simulink model "RC_Modelling"  (R2024a)
settings: Solver=FixedStepAuto  StartTime=0.0  StopTime=300  FixedStep=0.001  RelTol=1e-3
settings Model: Creator=devendra  LastModifiedBy=devendra

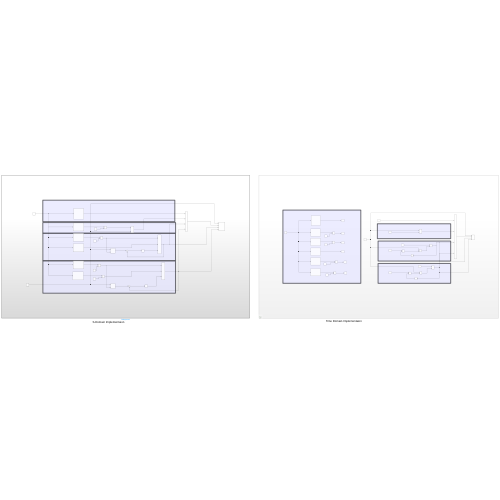
[thumbnail: Simulink's stored preview of the top-level diagram]
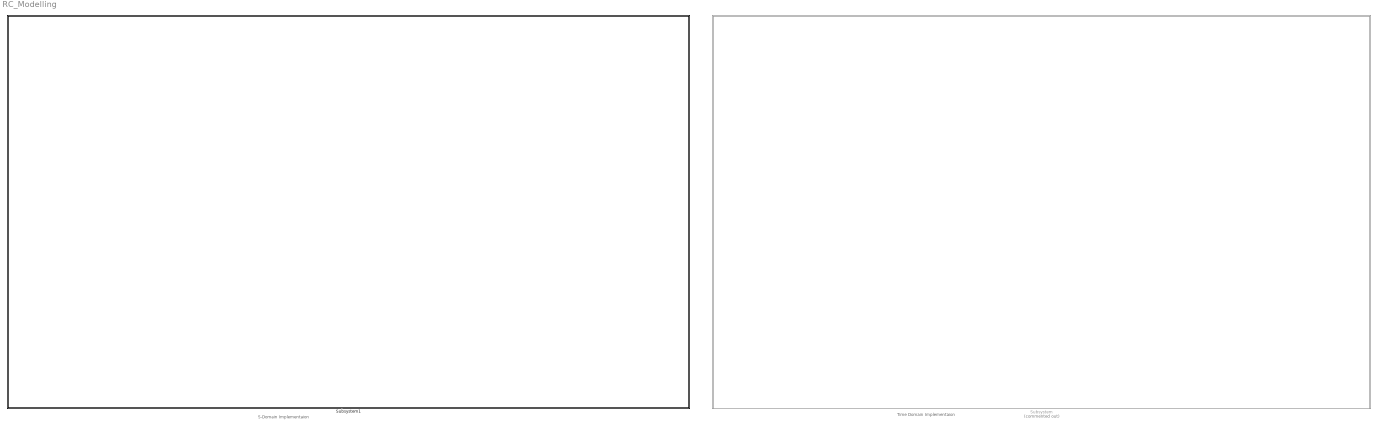
== system RC_Modelling ==
  note: Time Domain Implementaion
  note: S-Domain Implementaion
  Subsystem : Subsystem  Commented=on
  Subsystem1 : Subsystem

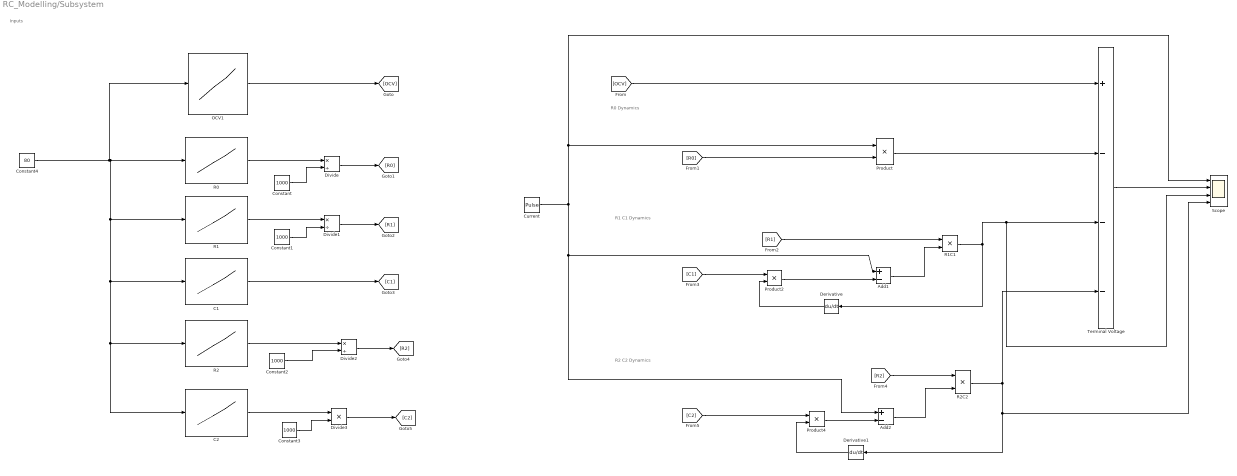
== system RC_Modelling/Subsystem ==
  note: Inputs
  note: R0 Dynamics
  note: R2 C2 Dynamics
  note: R1 C1 Dynamics
  Add1 : Sum  Inputs=+-
  Add2 : Sum  Inputs=+-
  C1 : Lookup_n-D  NumberOfTableDimensions=1  BreakpointsForDimension1=[0 5 10 20 30 40 50 60 70 80 90 100]  Table=[248 1482.7 2404.3 2466.7 2383.2 2193 2154.8 1498.3 1300.3 1714.9 1725.1 1840]  InternalRulePriority=Speed  RndMeth=Simplest
  C2 : Lookup_n-D  NumberOfTableDimensions=1  BreakpointsForDimension1=[0 5 10 20 30 40 50 60 70 80 90 100]  Table=[20.5 144.6 103 56.8 94.3 228 199.5 65.5 23.3 19.4 143 151]  InternalRulePriority=Speed  RndMeth=Simplest
  Constant{,1..3} (4 alike) : Constant  Value=1000
  Constant4 : Constant  Value=80
  Current : DiscretePulseGenerator  PulseType=Time based  Amplitude=5  Period=300  PulseWidth=25  SampleTime=100
  Derivative : Derivative
  Derivative1 : Derivative
  Divide : Product  Inputs=*/
  Divide1 : Product  Inputs=*/
  Divide2 : Product  Inputs=*/
  Divide3 : Product  Inputs=**
  OCV1 : Lookup_n-D  NumberOfTableDimensions=1  BreakpointsForDimension1=[0 5 10 15 20 30 40 50 60 70 80 90 95 100]  Table=[3.45 3.48 3.53 3.58 3.6 3.63 3.68 3.78 3.88 3.94 4.01 4.08 4.12 4.19]  InternalRulePriority=Speed  RndMeth=Simplest
  Product : Product
  Product2 : Product
  Product4 : Product
  R0 : Lookup_n-D  NumberOfTableDimensions=1  BreakpointsForDimension1=[0 5 10 20 30 40 50 60 70 80 90 100]  Table=[116.9 49 43.2 39.3 38.5 38.1 37.6 37.1 37 37.3 38.8 39]  InternalRulePriority=Speed  RndMeth=Simplest
  R1 : Lookup_n-D  NumberOfTableDimensions=1  BreakpointsForDimension1=[0 5 10 20 30 40 50 60 70 80 90 100]  Table=[67.5 22.6 21.6 25.8 22.4 20.2 21.6 22.2 19.8 20.8 23 23.7]  InternalRulePriority=Speed  RndMeth=Simplest
  "R1C1 " : Product
  R2 : Lookup_n-D  NumberOfTableDimensions=1  BreakpointsForDimension1=[0 5 10 20 30 40 50 60 70 80 90 100]  Table=[14.2 4.3 5.3 11.2 5.9 3.4 7.7 19 16.9 12.8 3.4 5]  InternalRulePriority=Speed  RndMeth=Simplest
  R2C2 : Product
  Scope : Scope  NumInputPorts=4
  Terminal Voltage : Sum  Inputs=+---
  wires:
  Product4/1 -> Add2/2
  Product/1 -> Terminal Voltage/2
  Add1/1 -> "R1C1 "/2
  "R1C1 "/1 -> Derivative/1, Scope/3, Terminal Voltage/3
  R2C2/1 -> Terminal Voltage/4, Scope/4, Derivative1/1
  Product2/1 -> Add1/2
  Current/1 -> Add2/1, Add1/1, Scope/1, Product/1
  [C1] -> Product2/1
  [R1] -> "R1C1 "/1
  Derivative/1 -> Product2/2
  [R2] -> R2C2/1
  Terminal Voltage/1 -> Scope/2
  Derivative1/1 -> Product4/2
  [C2] -> Product4/1
  [OCV] -> Terminal Voltage/1
  Add2/1 -> R2C2/2
  [R0] -> Product/2
  OCV1/1 -> [OCV]
  R0/1 -> Divide/1
  Constant/1 -> Divide/2
  R1/1 -> Divide1/1
  Constant1/1 -> Divide1/2
  Constant2/1 -> Divide2/2
  C2/1 -> Divide3/1
  Constant3/1 -> Divide3/2
  Divide/1 -> [R0]
  Divide1/1 -> [R1]
  C1/1 -> [C1]
  Divide2/1 -> [R2]
  Divide3/1 -> [C2]
  R2/1 -> Divide2/1
  Constant4/1 -> OCV1/1, C2/1, R2/1, C1/1, R1/1, R0/1

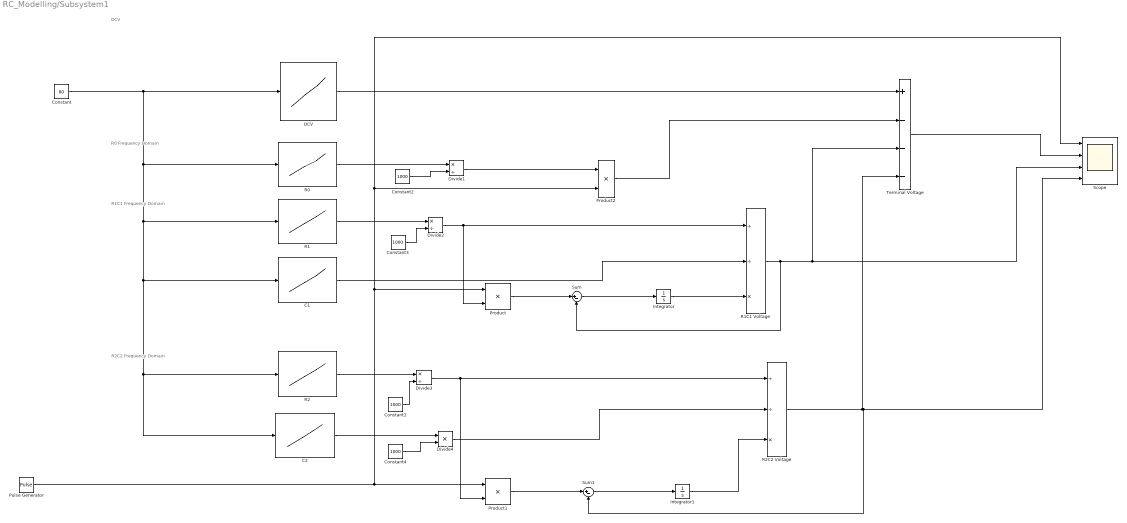
== system RC_Modelling/Subsystem1 ==
  note: R2C2 Frequency Domain
  note: R1C1 Frequency Domain
  note: R0 Frequency Domain
  note: OCV
  C1 : Lookup_n-D  NumberOfTableDimensions=1  BreakpointsForDimension1=[0 5 10 20 30 40 50 60 70 80 90 100]  Table=[248 1482.7 2404.3 2466.7 2383.2 2193 2154.8 1498.3 1300.3 1714.9 1725.1 1840]  InternalRulePriority=Speed  RndMeth=Simplest
  C2 : Lookup_n-D  NumberOfTableDimensions=1  BreakpointsForDimension1=[0 5 10 20 30 40 50 60 70 80 90 100]  Table=[20.5 144.6 103 56.8 94.3 228 199.5 65.5 23.3 19.4 143 151]  InternalRulePriority=Speed  RndMeth=Simplest
  Constant : Constant  Value=80
  Constant{1..4} (4 alike) : Constant  Value=1000
  Divide1 : Product  Inputs=*/
  Divide2 : Product  Inputs=*/
  Divide3 : Product  Inputs=*/
  Divide4 : Product  Inputs=**
  Integrator : Integrator
  Integrator1 : Integrator
  OCV : Lookup_n-D  NumberOfTableDimensions=1  BreakpointsForDimension1=[0 5 10 15 20 30 40 50 60 70 80 90 95 100]  Table=[3.45 3.48 3.53 3.58 3.6 3.63 3.68 3.78 3.88 3.94 4.01 4.08 4.12 4.19]  InternalRulePriority=Speed  RndMeth=Simplest
  Product : Product
  Product1 : Product
  Product2 : Product
  Pulse Generator : DiscretePulseGenerator  PulseType=Time based  Amplitude=5  Period=300  PulseWidth=25
  R0 : Lookup_n-D  NumberOfTableDimensions=1  BreakpointsForDimension1=[0 5 10 20 30 40 50 60 70 80 90 100]  Table=[116.9 49 43.2 39.3 38.5 38.1 37.6 37.1 37 37.3 38.8 39]  InternalRulePriority=Speed  RndMeth=Simplest
  R1 : Lookup_n-D  NumberOfTableDimensions=1  BreakpointsForDimension1=[0 5 10 20 30 40 50 60 70 80 90 100]  Table=[67.5 22.6 21.6 25.8 22.4 20.2 21.6 22.2 19.8 20.8 23 23.7]  InternalRulePriority=Speed  RndMeth=Simplest
  R1C1 Voltage : Product  Inputs=//*
  R2 : Lookup_n-D  NumberOfTableDimensions=1  BreakpointsForDimension1=[0 5 10 20 30 40 50 60 70 80 90 100]  Table=[14.2 4.3 5.3 11.2 5.9 3.4 7.7 19 16.9 12.8 3.4 5]  InternalRulePriority=Speed  RndMeth=Simplest
  R2C2 Voltage : Product  Inputs=//*
  Scope : Scope  NumInputPorts=4
  Sum : Sum  Inputs=|+-
  Sum1 : Sum  Inputs=|+-
  Terminal Voltage : Sum  Inputs=+---
  wires:
  Product/1 -> Sum/1
  Integrator1/1 -> R2C2 Voltage/3
  Constant/1 -> C2/1, R2/1, C1/1, R1/1, R0/1, OCV/1
  Pulse Generator/1 -> Scope/1, Product2/2, Product/1, Product1/1
  Integrator/1 -> R1C1 Voltage/3
  Product1/1 -> Sum1/1
  R2C2 Voltage/1 -> Scope/4, Sum1/2, Terminal Voltage/4
  R1C1 Voltage/1 -> Terminal Voltage/3, Scope/3, Sum/2
  Sum/1 -> Integrator/1
  Sum1/1 -> Integrator1/1
  Product2/1 -> Terminal Voltage/2
  Terminal Voltage/1 -> Scope/2
  C1/1 -> R1C1 Voltage/2
  OCV/1 -> Terminal Voltage/1
  Divide1/1 -> Product2/1
  R0/1 -> Divide1/1
  Constant2/1 -> Divide1/2
  R1/1 -> Divide2/1
  Divide2/1 -> Product/2, R1C1 Voltage/1
  Constant3/1 -> Divide2/2
  R2/1 -> Divide3/1
  Constant1/1 -> Divide3/2
  Divide3/1 -> Product1/2, R2C2 Voltage/1
  C2/1 -> Divide4/1
  Divide4/1 -> R2C2 Voltage/2
  Constant4/1 -> Divide4/2
